simulink model "hoverController"  (R2021b)
settings: Solver=VariableStepAuto  StartTime=0.0  StopTime=20  MaxStep=0.0002  MinStep=0.0001  RelTol=1e-3
values from neighbouring files (symbols this model uses):
  num = [0.25 * 0.07869]    [untitled.m]
undefined symbols (not defined in the file or in its folder): anal_den, anal_num, den, g, maxRotorLift, weight
settings Model: Creator=chris  LastModifiedBy=chris

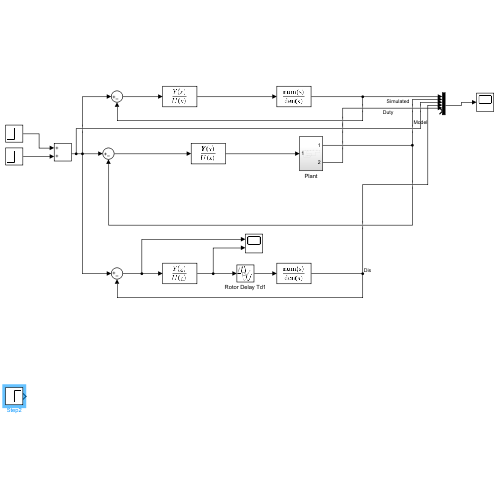
[thumbnail: Simulink's stored preview of the top-level diagram]
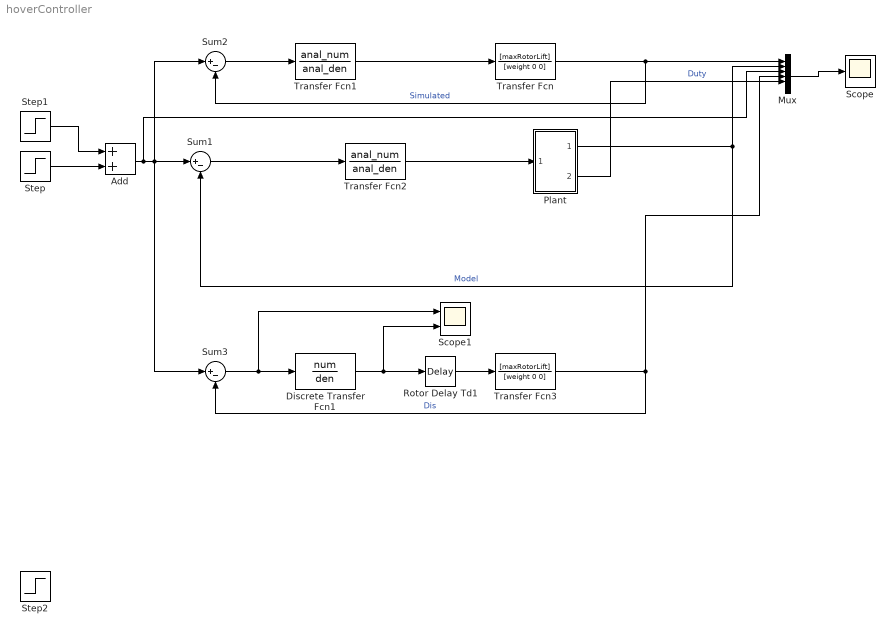
== system hoverController ==
  Add : Sum
  Discrete Transfer Fcn1 : DiscreteTransferFcn  Numerator=num  Denominator=den  SampleTime=t
  Mux : Mux  Inputs=6
  Plant : Subsystem
  Rotor Delay Td1 : TransportDelay  DelayTime=t
  Scope : Scope
  Scope1 : Scope  NumInputPorts=2
  Step : Step  SampleTime=0
  Step1 : Step  Time=5  After=0  SampleTime=0
  Step2 : Step  SampleTime=0
  Sum1 : Sum  Inputs=|+-
  Sum2 : Sum  Inputs=|+-
  Sum3 : Sum  Inputs=|+-
  Transfer Fcn : TransferFcn  Numerator=[maxRotorLift]  Denominator=[weight 0 0]
  Transfer Fcn1 : TransferFcn  Numerator=anal_num  Denominator=anal_den
  Transfer Fcn2 : TransferFcn  Numerator=anal_num  Denominator=anal_den
  Transfer Fcn3 : TransferFcn  Numerator=[maxRotorLift]  Denominator=[weight 0 0]
  wires:
  Step/1 -> Add/2
  Step1/1 -> Add/1
  Plant/1(Out1) -> Sum1/2, Mux/2  "Model"
  Sum1/1 -> Transfer Fcn2/1
  Sum2/1 -> Transfer Fcn1/1
  Transfer Fcn/1 -> Sum2/2, Mux/1  "Simulated"
  Mux/1 -> Scope/1
  Transfer Fcn1/1 -> Transfer Fcn/1
  Plant/2(Out2) -> Mux/5  "Duty"
  Transfer Fcn2/1 -> Plant/1(In1)
  Transfer Fcn3/1 -> Mux/4, Sum3/2  "Dis"
  Sum3/1 -> Scope1/1, Discrete Transfer Fcn1/1
  Discrete Transfer Fcn1/1 -> Scope1/2, Rotor Delay Td1/1
  Add/1 -> Mux/3, Sum3/1, Sum2/1, Sum1/1
  Rotor Delay Td1/1 -> Transfer Fcn3/1

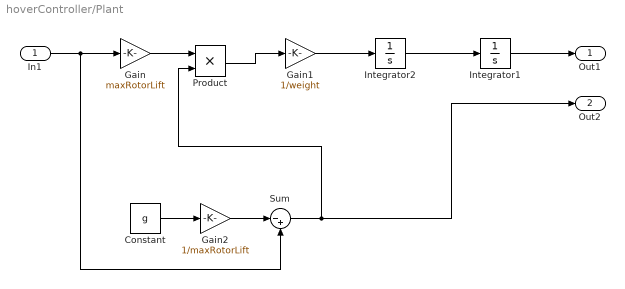
== system hoverController/Plant ==
  In1 : Inport
  Constant : Constant  Value=g
  Gain : Gain  Gain=maxRotorLift
  Gain1 : Gain  Gain=1/weight
  Gain2 : Gain  Gain=1/maxRotorLift
  Integrator1 : Integrator
  Integrator2 : Integrator
  Product : Product
  Sum : Sum  Inputs=|-+
  Out1 : Outport
  Out2 : Outport  Port=2
  wires:
  Gain/1 -> Product/1
  Integrator2/1 -> Integrator1/1
  Integrator1/1 -> Out1/1
  In1/1 -> Sum/2, Gain/1
  Constant/1 -> Gain2/1
  Gain1/1 -> Integrator2/1
  Gain2/1 -> Sum/1
  Sum/1 -> Product/2, Out2/1
  Product/1 -> Gain1/1
